simulink model "project_2_ic"  (R2012b)
settings: Solver=ode45  StartTime=0.0  StopTime=50  RelTol=1e-3
settings Model: Creator=neel  LastModifiedBy=neel

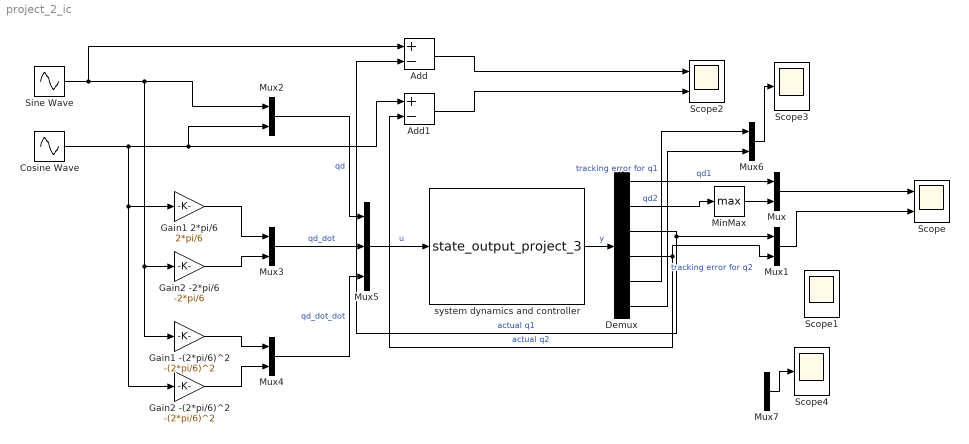
== system project_2_ic ==
  Add : Sum  Inputs=+-
  Add1 : Sum  Inputs=+-
  Cosine Wave : Sin  Amplitude=0.2  Frequency=2*pi/6  Phase=pi/2  SampleTime=0
  Demux : Demux  Outputs=6
  Gain1 -(2*pi/6)^2 : Gain  Gain=-(2*pi/6)^2
  Gain1 2*pi/6 : Gain  Gain=2*pi/6
  Gain2 -(2*pi/6)^2 : Gain  Gain=-(2*pi/6)^2
  Gain2 -2*pi/6 : Gain  Gain=-2*pi/6
  MinMax : MinMax  Function=max
  Mux{,1..4,6..7} (7 alike) : Mux  Inputs=2
  Mux5 : Mux  Inputs=3
  Scope : Scope  NumInputPorts=2
      settings: YMin=-5~-5  YMax=5~5
  Scope1 : Scope  NumInputPorts=2
      settings: TimeRange=0.1299083949579183  YMin=1.222459437991586e-05~-0.02  YMax=5.922333327175282e-05~0.1
  Scope2 : Scope  NumInputPorts=2
      settings: YMin=-5~-5  YMax=5~5  SaveName=ScopeData2
  Scope3 : Scope
      settings: TimeRange=0.1299083949579183  YMin=-0.19  YMax=0.03  SaveName=ScopeData3
  Scope4 : Scope
      settings: TimeRange=0.1299083949579183  YMin=1.22246e-05  YMax=5.92233e-05  SaveName=ScopeData4
  Sine Wave : Sin  Amplitude=0.2  Frequency=2*pi/6  SampleTime=0
  system dynamics and controller : S-Function  FunctionName=state_output_project_3  EnableBusSupport=off
  wires:
  system dynamics and controller/1 -> Demux/1  "y"
  Demux/1 -> Mux/1  "qd1"
  Demux/2 -> MinMax/1  "qd2"
  Demux/3 -> Mux1/1, Add/2  "actual q1"
  Demux/4 -> Mux1/2, Add1/2  "actual q2"
  ? -> Scope1/1  "tracking error for q1"
  ? -> Scope1/2  "tracking error for q2"
  Mux1/1 -> Scope/2
  Mux2/1 -> Mux5/1  "qd"
  Mux3/1 -> Mux5/2  "qd_dot"
  Mux4/1 -> Mux5/3  "qd_dot_dot"
  Sine Wave/1 -> Add/1, Gain1 -(2*pi/6)^2/1, Gain2 -2*pi/6/1, Mux2/1
  Cosine Wave/1 -> Add1/1, Mux2/2, Gain2 -(2*pi/6)^2/1, Gain1 2*pi/6/1
  Gain1 -(2*pi/6)^2/1 -> Mux4/1
  Gain2 -(2*pi/6)^2/1 -> Mux4/2
  Gain2 -2*pi/6/1 -> Mux3/2
  Gain1 2*pi/6/1 -> Mux3/1
  Mux5/1 -> system dynamics and controller/1  "u"
  Add/1 -> Scope2/1
  Add1/1 -> Scope2/2
  Demux/5 -> Mux6/1  "tracking error for q1"
  Demux/6 -> Mux6/2  "tracking error for q2"
  Mux6/1 -> Scope3/1
  Mux7/1 -> Scope4/1
  ? -> Mux7/1
  ? -> Mux7/2
  Mux/1 -> Scope/1
  MinMax/1 -> Mux/2
